simulink model "testbed_Radio"  (R2019b)
settings: Solver=ode113  StartTime=0.0  StopTime=7200  MaxStep=60  MinStep=1e-13  RelTol=1e-16  AbsTol=1e-16
model workspace (MAT data in the model file):
  mi = 1
values from neighbouring files (symbols this model uses):
  ParAltimeter = init_ParAltimeter()    [init_testbed.m]
  ParBody = init_ParBody()    [init_testbed.m]
  ParCamera = init_ParCamera()    [init_testbed.m]
  ParEphemerides = init_ParEphemerides()    [init_testbed.m]
  ParRadio = init_ParRadio()    [init_testbed.m]
  ParSpacecraft = init_ParSpacecraft()    [init_testbed.m]
settings Model: Creator=tomma  LastModifiedBy=antoniogenova

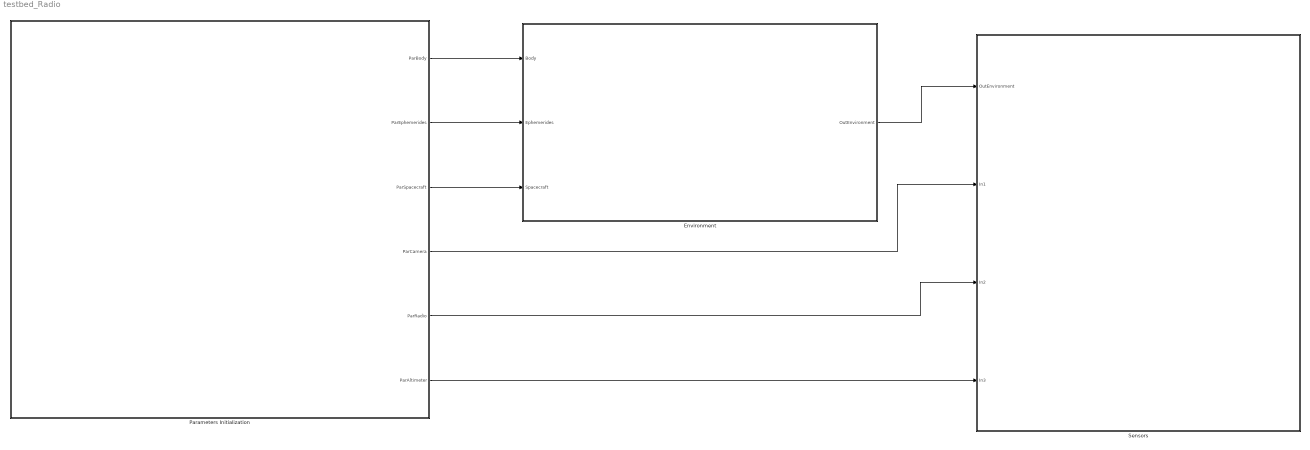
== system testbed_Radio ==
  Environment : Subsystem
  "Parameters Initialization " : Subsystem
  Sensors : Subsystem
  wires:
  "Parameters Initialization "/1(ParBody) -> Environment/1(Body)
  "Parameters Initialization "/2(ParEphemerides) -> Environment/2(Ephemerides)
  "Parameters Initialization "/3(ParSpacecraft) -> Environment/3(Spacecraft)
  Environment/1(OutEnvironment) -> Sensors/1(OutEnvironment)
  "Parameters Initialization "/4(ParCamera) -> Sensors/2(In1)
  "Parameters Initialization "/5(ParRadio) -> Sensors/3(In2)
  "Parameters Initialization "/6(ParAltimeter) -> Sensors/4(In3)

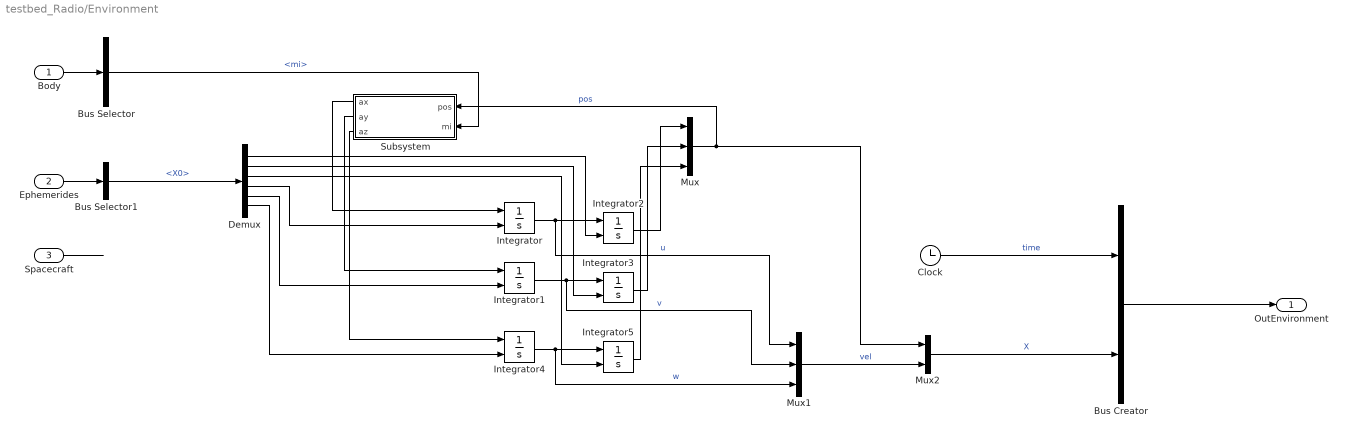
== system testbed_Radio/Environment ==
  Body : Inport
  Ephemerides : Inport  Port=2
  Spacecraft : Inport  Port=3
  Bus Creator : BusCreator  Inputs=2
  Bus Selector : BusSelector  OutputSignals=ParBody_Bus.mi
  Bus Selector1 : BusSelector  OutputSignals=ParEphemerides_Bus.X0
  Clock : Clock
  Demux : Demux  Outputs=6
  Integrator{,1..5} (6 alike) : Integrator  InitialConditionSource=external  ContinuousStateAttributes="\"\""
  Mux : Mux  Inputs=3
  Mux1 : Mux  Inputs=3
  Mux2 : Mux  Inputs=2
  Subsystem : Subsystem
  OutEnvironment : Outport
  wires:
  Integrator1/1 -> Mux1/2, Integrator3/1  "v"
  Clock/1 -> Bus Creator/1  "time"
  Bus Creator/1 -> OutEnvironment/1
  Integrator4/1 -> Mux1/3, Integrator5/1  "w"
  Subsystem/3(az) -> Integrator4/1
  Integrator2/1 -> Mux/1
  Demux/2 -> Integrator3/2
  Demux/3 -> Integrator5/2
  Mux2/1 -> Bus Creator/2  "X"
  Subsystem/2(ay) -> Integrator1/1
  Integrator3/1 -> Mux/2
  Mux/1 -> Mux2/1, Subsystem/1(pos)  "pos"
  Integrator5/1 -> Mux/3
  Demux/6 -> Integrator4/2
  Demux/1 -> Integrator2/2
  Integrator/1 -> Mux1/1, Integrator2/1  "u"
  Mux1/1 -> Mux2/2  "vel"
  Subsystem/1(ax) -> Integrator/1
  Demux/4 -> Integrator/2
  Demux/5 -> Integrator1/2
  Bus Selector1/1 -> Demux/1  "<X0>"
  Body/1 -> Bus Selector/1
  Ephemerides/1 -> Bus Selector1/1
  Bus Selector/1 -> Subsystem/2(mi)  "<mi>"
  Spacecraft/1 -> ?

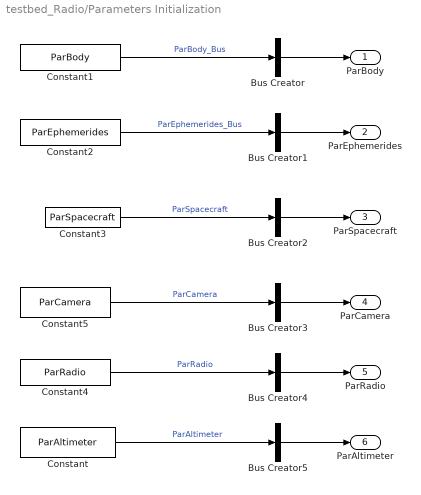
== system testbed_Radio/Parameters Initialization  ==
  Bus Creator{,1..5} (6 alike) : BusCreator  Inputs=1
  Constant : Constant  Value=ParAltimeter  OutDataTypeStr=Bus: ParAltimeter_Bus
  Constant1 : Constant  Value=ParBody  OutDataTypeStr=Bus: ParBody_Bus
  Constant2 : Constant  Value=ParEphemerides  OutDataTypeStr=Bus: ParEphemerides_Bus
  Constant3 : Constant  Value=ParSpacecraft  OutDataTypeStr=Bus: ParSpacecraft_Bus
  Constant4 : Constant  Value=ParRadio  OutDataTypeStr=Bus: ParRadio_Bus
  Constant5 : Constant  Value=ParCamera  OutDataTypeStr=Bus: ParCamera_Bus
  ParBody : Outport
  ParEphemerides : Outport  Port=2
  ParSpacecraft : Outport  Port=3
  ParCamera : Outport  Port=4
  ParRadio : Outport  Port=5
  ParAltimeter : Outport  Port=6
  wires:
  Constant/1 -> Bus Creator5/1  "ParAltimeter"
  Constant5/1 -> Bus Creator3/1  "ParCamera"
  Constant4/1 -> Bus Creator4/1  "ParRadio"
  Constant1/1 -> Bus Creator/1  "ParBody_Bus"
  Constant2/1 -> Bus Creator1/1  "ParEphemerides_Bus"
  Constant3/1 -> Bus Creator2/1  "ParSpacecraft"
  Bus Creator/1 -> ParBody/1
  Bus Creator1/1 -> ParEphemerides/1
  Bus Creator2/1 -> ParSpacecraft/1
  Bus Creator3/1 -> ParCamera/1
  Bus Creator4/1 -> ParRadio/1
  Bus Creator5/1 -> ParAltimeter/1

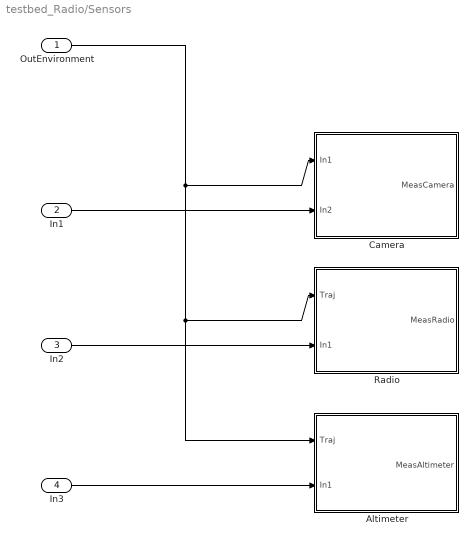
== system testbed_Radio/Sensors ==
  OutEnvironment : Inport
  In1 : Inport  Port=2
  In2 : Inport  Port=3
  In3 : Inport  Port=4
  Altimeter : Subsystem
  Camera : Subsystem
  Radio : Subsystem
  wires:
  OutEnvironment/1 -> Camera/1(In1), Altimeter/1(Traj), Radio/1(Traj)
  In1/1 -> Camera/2(In2)
  In2/1 -> Radio/2(In1)
  In3/1 -> Altimeter/2(In1)

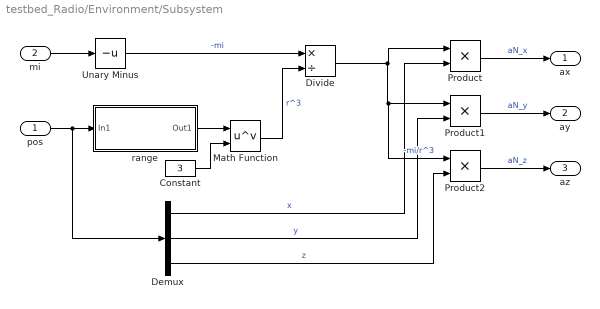
== system testbed_Radio/Environment/Subsystem ==
  pos : Inport
  mi : Inport  Port=2
  Constant : Constant  Value=3
  Demux : Demux  Outputs=3
  Divide : Product  Inputs=*/
  Math Function : Math  Operator=pow  SignedPower=off  SaturateOnIntegerOverflow=on
  Product : Product
  Product1 : Product
  Product2 : Product
  Unary Minus : UnaryMinus
  range : Subsystem
  ax : Outport
  ay : Outport  Port=2
  az : Outport  Port=3
  wires:
  pos/1 -> Demux/1, range/1(In1)
  mi/1 -> Unary Minus/1
  Unary Minus/1 -> Divide/1  "-mi"
  Constant/1 -> Math Function/2
  range/1(Out1) -> Math Function/1
  Math Function/1 -> Divide/2  "r^3"
  Divide/1 -> Product2/1, Product1/1, Product/1  "-mi/r^3"
  Demux/1 -> Product/2  "x"
  Demux/2 -> Product1/2  "y"
  Demux/3 -> Product2/2  "z"
  Product/1 -> ax/1  "aN_x"
  Product1/1 -> ay/1  "aN_y"
  Product2/1 -> az/1  "aN_z"

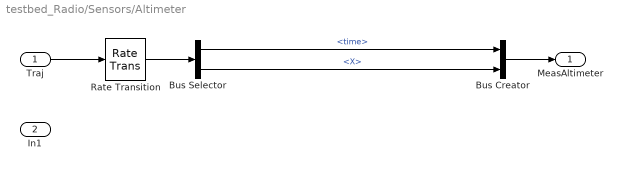
== system testbed_Radio/Sensors/Altimeter ==
  Traj : Inport
  In1 : Inport  Port=2
  Bus Creator : BusCreator  Inputs=2
  Bus Selector : BusSelector  OutputSignals=time,X
  Rate Transition : RateTransition  OutPortSampleTime=ParAltimeter.countime
  MeasAltimeter : Outport
  wires:
  Traj/1 -> Rate Transition/1
  Bus Selector/2 -> Bus Creator/2  "<X>"
  Bus Selector/1 -> Bus Creator/1  "<time>"
  Bus Creator/1 -> MeasAltimeter/1
  Rate Transition/1 -> Bus Selector/1

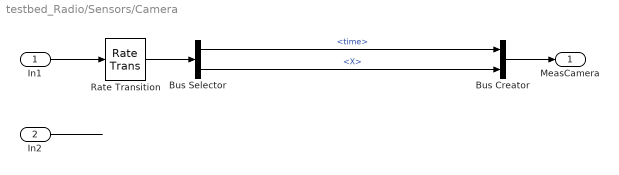
== system testbed_Radio/Sensors/Camera ==
  In1 : Inport
  In2 : Inport  Port=2
  Bus Creator : BusCreator  Inputs=2
  Bus Selector : BusSelector  OutputSignals=time,X
  Rate Transition : RateTransition  OutPortSampleTime=ParCamera.countime
  MeasCamera : Outport
  wires:
  In1/1 -> Rate Transition/1
  Bus Creator/1 -> MeasCamera/1
  Bus Selector/2 -> Bus Creator/2  "<X>"
  Rate Transition/1 -> Bus Selector/1
  Bus Selector/1 -> Bus Creator/1  "<time>"
  In2/1 -> ?

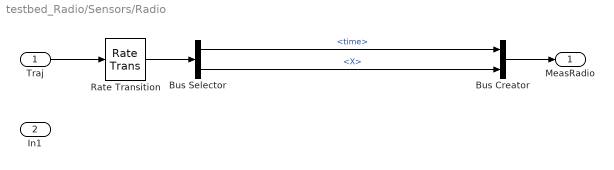
== system testbed_Radio/Sensors/Radio ==
  Traj : Inport
  In1 : Inport  Port=2
  Bus Creator : BusCreator  Inputs=2
  Bus Selector : BusSelector  OutputSignals=time,X
  Rate Transition : RateTransition  OutPortSampleTime=ParRadio.countime
  MeasRadio : Outport
  wires:
  Rate Transition/1 -> Bus Selector/1
  Bus Selector/1 -> Bus Creator/1  "<time>"
  Traj/1 -> Rate Transition/1
  Bus Creator/1 -> MeasRadio/1
  Bus Selector/2 -> Bus Creator/2  "<X>"

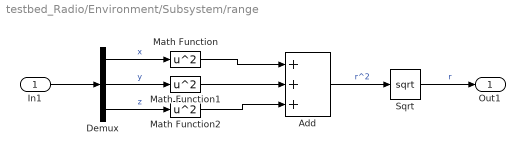
== system testbed_Radio/Environment/Subsystem/range ==
  In1 : Inport
  Add : Sum  Inputs=+++
  Demux : Demux  Outputs=3
  Math Function : Math  Operator=square  SignedPower=off  SaturateOnIntegerOverflow=on
  Math Function1 : Math  Operator=square  SignedPower=off  SaturateOnIntegerOverflow=on
  Math Function2 : Math  Operator=square  SignedPower=off  SaturateOnIntegerOverflow=on
  Sqrt : Sqrt  SaturateOnIntegerOverflow=on
  Out1 : Outport
  wires:
  In1/1 -> Demux/1
  Demux/1 -> Math Function/1  "x"
  Demux/2 -> Math Function1/1  "y"
  Demux/3 -> Math Function2/1  "z"
  Math Function/1 -> Add/1
  Math Function1/1 -> Add/2
  Math Function2/1 -> Add/3
  Add/1 -> Sqrt/1  "r^2"
  Sqrt/1 -> Out1/1  "r"
